simulink model "PubIfDecisionTOS_MDL"  (R2020b)
settings: configuration reference "DspaceConfig" (kept outside this file)
PostLoadFcn:
  | if any(exist('dsrtsu_mdlpostloadfcn', 'file') ~= 0), dsrtsu_mdlpostloadfcn('Execute', bdroot); end
InitFcn:
  | , if any(exist('dsmpb_private', 'file') ~= 0), dsmpb_private('dsmpb_mdlclblib', 'Init', bdroot); end,
undefined symbols (not defined in the file or in its folder): C_TOS_ACCEgoRAxletoFbumplength_m, C_TOS_ACCTargetFront_Flag, C_TOS_AEBJAPedObjDxThre_Val, C_TOS_AEBJAPedObjDyThre_Val, C_TOS_AEBJATargetSize_Val, C_TOS_AEBJAVehObjDxThre_Val, C_TOS_AEBJAVehObjDyThre_Val, C_TOS_AEBJuncPedTargetSize_Val, C_TOS_AEBLatObjDxThre_Val, C_TOS_AEBLatPedDyThre_Val, C_TOS_AEBLatTargetSize_Val, C_TOS_AEBLongTargetInEgoFront_Flag, C_TOS_axAbsGround_Parameter, C_TOS_CameraConfirmedFlag, C_TOS_CNsubjWidth, C_TOS_CurrentLaneCoreMinWidth_Val, C_TOS_CutInProb_Val_Zero, C_TOS_CutOutProb_Val_Zero, C_TOS_D2R_Val, C_TOS_DefaultValueObjectToCenterLine_dy, C_TOS_EgoCarWidth_Val, C_TOS_EgoDxRefPoint_m, C_TOS_EgoRAxletoFbumplength_m, C_TOS_HalfWidthVehicle_Con, C_TOS_HWA_CurrentLaneFlag, C_TOS_HWA_LeftLaneFlag, C_TOS_HWA_MovingDir_Vaild, C_TOS_HWA_MovState_Vaild, C_TOS_HWA_RightLaneFlag, C_TOS_LaneLineCourseErrorFront, C_TOS_LaneLineCourseErrorRear, C_TOS_MotorbikeDefaultWidth_m, C_TOS_NumberOfEffectiveTargets, C_TOS_Obj_Age_Val, C_TOS_Objdx_Constraint_Val, C_TOS_ObjectDefaultWidth_m, C_TOS_ObjInCurrentLane_Val, C_TOS_ObjInCurrentLaneValid, C_TOS_ObjInLeftLaneValid, C_TOS_ObjInRightLaneValid, C_TOS_ObjNotInCurrentLane_Val, C_TOS_ObjNotREElementType, C_TOS_ObjPredictDis_dy_ConstantVal_Zeros, C_TOS_ObjToCenterLine_ConstantVal_Zeros, C_TOS_OFMObjIDInvilad_Val, C_TOS_PIL_LatDisCons_Val_zero, C_TOS_PIL_ObjectCutInFlag_b, C_TOS_PIL_ObjectCutOutFlag_b, C_TOS_PIL_ObjLaneProb_al_Val, C_TOS_PP_ObjFusType_FC_Confirm_b, C_TOS_PP_ObjFusType_FC_FR_Confirm_b, C_TOS_PP_ObjFusType_FR_Confirm_b, C_TOS_RE_80BoolDefault_Val, C_TOS_RE_80Single181Default_Val, C_TOS_RE_80Single255Default_Val, C_TOS_RE_80Uint8Default_Val, C_TOS_RE_D2R, C_TOS_RE_D_180_Val, C_TOS_RE_InvalidObjectID_Val, C_TOS_RE_InvalidTargetChainDir_Val ... (+142)
libraries: simulink x1650, TOS_LIB x361, canfdmsglib x14
(part 33 of 69)

== system PubIfDecisionTOS_MDL/TOS_20201112/TOS_2012080320/PIL_1029/ObjCutInOut_Prob/ObjectCutOut/CutOutProb_Calculate/CutOutProb_Calculate/CutOutPredictDis_dy/CutOutPredictTime_Constraint2 ==
  note: 压线行驶
  note: 目标由右→左；过线
  note: 当前距离dy + 预测距离dy'
  note: 预测距离dy'
  note: 目标由左→右；过线
  ObjectToCenterLine_dy : Inport
  PredictTimeConstraint : Inport  Port=2
  PP_ObjectToCenterLine_vyc : Inport  Port=3
  Object_VY : Inport  Port=4
  Add3 : Sum  OutDataTypeStr=single
  Compare To Constant : simulink/Logic and Bit Operations/Compare To Constant  relop=<  const=C_TOS_ObjToCenterLine_ConstantVal_Zeros  OutDataTypeStr=boolean
      settings: AttributesFormatString=C_TOS_ObjToCenterLine_ConstantVal_Zeros = 0
  Compare To Constant1 : simulink/Logic and Bit Operations/Compare To Constant  relop=>  const=C_TOS_ObjToCenterLine_ConstantVal_Zeros  OutDataTypeStr=boolean
      settings: AttributesFormatString=C_TOS_ObjToCenterLine_ConstantVal_Zeros = 0
  Compare To Constant2 : simulink/Logic and Bit Operations/Compare To Constant  relop=>  const=C_TOS_ObjToCenterLine_ConstantVal_Zeros  OutDataTypeStr=boolean
      settings: AttributesFormatString=C_TOS_ObjToCenterLine_ConstantVal_Zeros = 0
  Compare To Constant3 : simulink/Logic and Bit Operations/Compare To Constant  relop=<  const=C_TOS_ObjToCenterLine_ConstantVal_Zeros  OutDataTypeStr=boolean
      settings: AttributesFormatString=C_TOS_ObjToCenterLine_ConstantVal_Zeros = 0
  Compare To Constant4 : simulink/Logic and Bit Operations/Compare To Constant  relop===  const=C_TOS_ObjToCenterLine_ConstantVal_Zeros  OutDataTypeStr=boolean
      settings: AttributesFormatString=C_TOS_ObjToCenterLine_ConstantVal_Zeros = 0
  Compare To Constant5 : simulink/Logic and Bit Operations/Compare To Constant  relop=>=  const=P_TOS_CutoutObjvyThre  OutDataTypeStr=boolean
      settings: AttributesFormatString=P_TOS_CutoutObjvyThre = 0.3
  Constant : Constant  Value=0  OutDataTypeStr=single
  Constant2 : Constant  Value=C_TOS_ObjPredictDis_dy_ConstantVal_Zeros  OutDataTypeStr=single
      settings: AttributesFormatString=C_TOS_ObjPredictDis_dy_ConstantVal_Zeros = 0
  Constant5 : Constant  Value=C_TOS_ObjPredictDis_dy_ConstantVal_Zeros  OutDataTypeStr=single
      settings: AttributesFormatString=C_TOS_ObjPredictDis_dy_ConstantVal_Zeros = 0
  Constant6 : Constant  Value=C_TOS_ObjPredictDis_dy_ConstantVal_Zeros  OutDataTypeStr=single
      settings: AttributesFormatString=C_TOS_ObjPredictDis_dy_ConstantVal_Zeros = 0
  Divide4 : Product  Inputs=**  OutDataTypeStr=single
  Logical Operator3 : Logic  AllPortsSameDT=off  OutDataTypeStr=boolean
  Logical Operator4 : Logic  AllPortsSameDT=off  OutDataTypeStr=boolean
  Switch : Switch  Criteria=u2 > Threshold
  Switch3 : Switch  Criteria=u2 > Threshold  OutDataTypeStr=single
  Switch4 : Switch  Criteria=u2 > Threshold  OutDataTypeStr=single
  Switch5 : Switch  Criteria=u2 > Threshold  OutDataTypeStr=single
  CutOutPredictDis_dy : Outport  OutDataTypeStr=single
  wires:
  Constant/1 -> Switch/3
  Switch/1 -> Divide4/2
  Compare To Constant5/1 -> Switch/2
  Object_VY/1 -> Compare To Constant5/1
  PP_ObjectToCenterLine_vyc/1 -> Switch/1
  PredictTimeConstraint/1 -> Divide4/1
  Switch4/1 -> Switch3/3
  Compare To Constant2/1 -> Logical Operator4/1
  [ObjectToCenterLine_dy] -> Compare To Constant1/1
  Constant6/1 -> Switch4/1
  Compare To Constant1/1 -> Logical Operator3/2
  Switch5/1 -> Switch4/3
  Constant2/1 -> Switch3/1
  Compare To Constant4/1 -> Switch5/2
  Switch3/1 -> CutOutPredictDis_dy/1
  [ObjectToCenterLine_dy] -> Compare To Constant3/1
  Compare To Constant3/1 -> Logical Operator4/2
  [ObjectToCenterLine_dy] -> Compare To Constant4/1
  ObjectToCenterLine_dy/1 -> Add3/2, [ObjectToCenterLine_dy]
  Divide4/1 -> Add3/1
  Logical Operator4/1 -> Switch4/2
  Add3/1 -> Switch5/3, Compare To Constant2/1, Compare To Constant/1
  Constant5/1 -> Switch5/1
  Logical Operator3/1 -> Switch3/2
  Compare To Constant/1 -> Logical Operator3/1

== system PubIfDecisionTOS_MDL/TOS_20201112/TOS_2012080320/PIL_1029/ObjCutInOut_Prob/ObjectCutOut/CutOutProb_Calculate/CutOutProb_Calculate/CutOutProb/CutOutObjWidthConstraint ==
  note: 根据目标宽度，修正CutOut预测距离（左右车辆边缘）
  note: 目标在中心线左侧
  note: 目标在中心线右侧
  CutOutPredictDis_dy : Inport  OutDataTypeStr=single
  PIL_ObjectToCenterLine_dy_Filt : Inport  Port=2  OutDataTypeStr=single
  Object_Width : Inport  Port=3
  ObjectType : Inport  Port=4
  Add : Sum
  Add1 : Sum  Inputs=+-
  C_HalfWidthVehicle_Con : Constant  Value=C_TOS_HalfWidthVehicle_Con  OutDataTypeStr=single
      settings: AttributesFormatString=C_TOS_HalfWidthVehicle_Con = 0.5
  Constant3 : Constant  Value=C_TOS_ObjToCenterLine_ConstantVal_Zeros  OutDataTypeStr=single
      settings: AttributesFormatString=C_TOS_ObjToCenterLine_ConstantVal_Zeros = 0
  Max : MinMax  Function=max  Inputs=2  OutDataTypeStr=single
  Max1 : MinMax  Inputs=2  OutDataTypeStr=single
  ObjectWidth_Check : Subsystem
  Product : Product  OutDataTypeStr=single
  Relational Operator : RelationalOperator  Operator=>  OutDataTypeStr=boolean  RndMeth=Nearest
  Switch : Switch  Criteria=u2 > Threshold  OutDataTypeStr=single
  constant1 : Constant  Value=0  OutDataTypeStr=single
  constant2 : Constant  Value=0  OutDataTypeStr=single
  CutOutPredictDis_dy_ObjWidthConstraint : Outport
  wires:
  ObjectType/1 -> ObjectWidth_Check/1(ObjectType)
  Object_Width/1 -> ObjectWidth_Check/2(Object_Width)
  ObjectWidth_Check/1(ObjectWidth) -> Product/2
  Add1/1 -> Max1/2
  Product/1 -> Add/1, Add1/2
  C_HalfWidthVehicle_Con/1 -> Product/1
  Relational Operator/1 -> Switch/2
  PIL_ObjectToCenterLine_dy_Filt/1 -> Relational Operator/1
  Constant3/1 -> Relational Operator/2
  constant1/1 -> Max/1
  CutOutPredictDis_dy/1 -> Add/2, Add1/1
  Max/1 -> Switch/1
  constant2/1 -> Max1/1
  Max1/1 -> Switch/3
  Add/1 -> Max/2
  Switch/1 -> CutOutPredictDis_dy_ObjWidthConstraint/1

== system PubIfDecisionTOS_MDL/TOS_20201112/TOS_2012080320/PIL_1029/ObjCutInOut_Prob/ObjectCutOut/CutOutProb_Calculate/CutOutProb_Calculate/CutOutProb/CutOutProb_Calculation ==
  note: 当前值 + 预测值 ；
  note: 预测时机修正
  CutOutPredictDis_dy_ObjWidthConstraint : Inport
  PIL_ObjectToCenterLine_dy_Filt : Inport  Port=2  OutDataTypeStr=single
  Abs : Abs
  Abs1 : Abs
  Add1 : Sum  Inputs=+-  OutDataTypeStr=single
  Add2 : Sum  Inputs=+-  OutDataTypeStr=single
  Compare To Constant1 : simulink/Logic and Bit Operations/Compare To Constant  relop=>=  const=P_TOS_CutOutMaxPredict_dy_Val  OutDataTypeStr=boolean
      settings: AttributesFormatString=P_TOS_CutOutMaxPredict_dy_Val = 2.8
  Compare To Constant2 : simulink/Logic and Bit Operations/Compare To Constant  relop=<=  const=P_TOS_CutOutMinPredict_dy_Val  OutDataTypeStr=boolean
      settings: AttributesFormatString=P_TOS_CutOutMinPredict_dy_Val = 1.5
  Divide1 : Product  Inputs=*/  OutDataTypeStr=single
  K_CutInMaxPredict_dy_Val : Constant  Value=P_TOS_CutOutMaxPredict_dy_Val  OutDataTypeStr=single
      settings: AttributesFormatString=P_TOS_CutOutMaxPredict_dy_Val = 2.8
  K_CutInMaxPredict_dy_Val1 : Constant  Value=P_TOS_CutOutMaxPredict_LatDis_Val  OutDataTypeStr=single
      settings: AttributesFormatString=P_TOS_CutOutMaxPredict_LatDis_Val = 2.8
  K_CutInMinPredict_dy_Val : Constant  Value=P_TOS_CutOutMinPredict_dy_Val  OutDataTypeStr=single
      settings: AttributesFormatString="P_TOS_CutOutMinPredict_dy_Val  = 1.5"
  Relational Operator1 : RelationalOperator  OutDataTypeStr=boolean  RndMeth=Nearest
  Switch1 : Switch  Criteria=u2 > Threshold
  Switch2 : Switch  Criteria=u2 > Threshold
  Switch3 : Switch  Criteria=u2 ~= 0
  CutOutProb_Calculation : Outport
  wires:
  Divide1/1 -> CutOutProb_Calculation/1
  Add2/1 -> Divide1/2
  Add1/1 -> Divide1/1
  [K_CutOutMinPredict_dy_Val] -> Add1/1
  CutOutPredictDis_dy_ObjWidthConstraint/1 -> Abs/1
  Switch2/1 -> Switch1/3
  K_CutInMaxPredict_dy_Val/1 -> [K_CutOutMaxPredict_dy_Val], Switch2/1
  Switch1/1 -> Switch3/3
  [K_CutOutMinPredict_dy_Val] -> Add2/1
  [K_CutOutMaxPredict_dy_Val] -> Add2/2
  K_CutInMinPredict_dy_Val/1 -> Switch1/1, [K_CutOutMinPredict_dy_Val]
  Compare To Constant2/1 -> Switch1/2
  Compare To Constant1/1 -> Switch2/2
  Abs/1 -> Switch2/3, Compare To Constant1/1, Compare To Constant2/1
  PIL_ObjectToCenterLine_dy_Filt/1 -> Abs1/1
  K_CutInMaxPredict_dy_Val1/1 -> Relational Operator1/2
  Relational Operator1/1 -> Switch3/2
  [K_CutOutMinPredict_dy_Val] -> Switch3/1
  Switch3/1 -> Add1/2
  Abs1/1 -> Relational Operator1/1

== system PubIfDecisionTOS_MDL/TOS_20201112/TOS_2012080320/PIL_1029/ObjCutInOut_Prob/ObjectCutOut/CutOutProb_Calculate/CutOutProb_Calculate/CutOutProb_ScopeConstraint/ObjectCutoutMind ==
  PIL_ObjectToCenterLine_dy_Filt : Inport
  PP_ObjectToCenterLine_vyc : Inport  Port=2  OutDataTypeStr=single
  PP_ObjectToCenterLine_dy : Inport  Port=3  OutDataTypeStr=single
  Object_Width : Inport  Port=4
  ObjectType : Inport  Port=5
  Abs1 : Abs
  Abs2 : Abs
  Compare To Constant1 : simulink/Logic and Bit Operations/Compare To Constant  relop=>  const=2.1  OutDataTypeStr=boolean
      settings: AttributesFormatString=P_TOS_CutoutObjvyThre_Val = 0.1
  Compare To Constant2 : simulink/Logic and Bit Operations/Compare To Constant  relop=<=  const=P_TOS_CutoutObjvyThre_Val  OutDataTypeStr=boolean
      settings: AttributesFormatString=P_TOS_CutoutObjvyThre_Val = 0.1
  CutOutObjCutinMov : Subsystem
  CutOutObjWidthConstraint : Subsystem
  Logical Operator1 : Logic  Operator=OR  Inputs=3  AllPortsSameDT=off  OutDataTypeStr=boolean
  Terminator : Terminator
  ObjectCutoutMindFlg : Outport
  ObjectCutoutMindFlg1 : Outport  Port=2
  ObjectCutoutMindFlg2 : Outport  Port=3
  ObjectCutoutMindFlg3 : Outport  Port=4
  wires:
  ObjectType/1 -> CutOutObjWidthConstraint/3(ObjectType)
  Compare To Constant1/1 -> Terminator/1
  Abs2/1 -> Compare To Constant1/1
  PIL_ObjectToCenterLine_dy_Filt/1 -> Abs2/1
  CutOutObjWidthConstraint/1(CutOutPredictDis_dy_ObjWidthConstraint) -> ObjectCutoutMindFlg3/1, Logical Operator1/3
  Logical Operator1/1 -> ObjectCutoutMindFlg/1
  PP_ObjectToCenterLine_dy/1 -> CutOutObjWidthConstraint/1(PP_ObjectToCenterLine_dy), CutOutObjCutinMov/2(ObjectToCenterLine_dy)
  PP_ObjectToCenterLine_vyc/1 -> CutOutObjCutinMov/1(PP_ObjectToCenterLine_vyc), Abs1/1
  Abs1/1 -> Compare To Constant2/1
  Object_Width/1 -> CutOutObjWidthConstraint/2(Object_Width)
  CutOutObjCutinMov/1(CutOutObjCutinMovflg) -> ObjectCutoutMindFlg2/1, Logical Operator1/2
  Compare To Constant2/1 -> ObjectCutoutMindFlg1/1, Logical Operator1/1

== system PubIfDecisionTOS_MDL/TOS_20201112/TOS_2012080320/PIL_1029/ProbCalculat/ProbCalculat/Subsystem/PIL_EgoVehiclePro/EgoVehicle_EgoLaneProb/Data1 ==
  Prob : Inport
  Bus Creator : BusCreator  Inputs=2
  Bus Creator1 : BusCreator  Inputs=2
  Compare To Constant10 : simulink/Logic and Bit Operations/Compare To Constant  relop=>=  const=0.001  OutDataTypeStr=boolean
  Constant1 : Constant  Value=0  OutDataTypeStr=single
  Constant2 : Constant  OutDataTypeStr=uint8
  Constant3 : Constant  Value=0  OutDataTypeStr=uint8
  Switch10 : Switch  Criteria=u2 > Threshold
  Out_Prob1 : Outport
  wires:
  Prob/1 -> Bus Creator/2, Compare To Constant10/1  "Prob1"
  Bus Creator/1 -> Switch10/1
  Bus Creator1/1 -> Switch10/3
  Constant2/1 -> Bus Creator/1  "Count1"
  Switch10/1 -> Out_Prob1/1  "Out_Prob1"
  Constant1/1 -> Bus Creator1/2  "Prob1"
  Constant3/1 -> Bus Creator1/1  "Count1"
  Compare To Constant10/1 -> Switch10/2

== system PubIfDecisionTOS_MDL/TOS_20201112/TOS_2012080320/PIL_1029/ProbCalculat/ProbCalculat/Subsystem/PIL_EgoVehiclePro/EgoVehicle_EgoLaneProb/Data10 ==
  Prob : Inport
  Bus Creator : BusCreator  Inputs=2
  Bus Creator1 : BusCreator  Inputs=2
  Compare To Constant10 : simulink/Logic and Bit Operations/Compare To Constant  relop=>=  const=0.001  OutDataTypeStr=boolean
  Constant1 : Constant  Value=0  OutDataTypeStr=single
  Constant2 : Constant  OutDataTypeStr=uint8
  Constant3 : Constant  Value=0  OutDataTypeStr=uint8
  Switch10 : Switch  Criteria=u2 > Threshold
  Out_Prob10 : Outport
  wires:
  Prob/1 -> Bus Creator/2, Compare To Constant10/1  "Prob10"
  Bus Creator/1 -> Switch10/1
  Bus Creator1/1 -> Switch10/3
  Constant2/1 -> Bus Creator/1  "Count10"
  Switch10/1 -> Out_Prob10/1  "Out_Prob10"
  Constant1/1 -> Bus Creator1/2  "Prob10"
  Constant3/1 -> Bus Creator1/1  "Count10"
  Compare To Constant10/1 -> Switch10/2

== system PubIfDecisionTOS_MDL/TOS_20201112/TOS_2012080320/PIL_1029/ProbCalculat/ProbCalculat/Subsystem/PIL_EgoVehiclePro/EgoVehicle_EgoLaneProb/Data2 ==
  Prob : Inport
  Bus Creator : BusCreator  Inputs=2
  Bus Creator1 : BusCreator  Inputs=2
  Compare To Constant10 : simulink/Logic and Bit Operations/Compare To Constant  relop=>=  const=0.001  OutDataTypeStr=boolean
  Constant1 : Constant  Value=0  OutDataTypeStr=single
  Constant2 : Constant  OutDataTypeStr=uint8
  Constant3 : Constant  Value=0  OutDataTypeStr=uint8
  Switch10 : Switch  Criteria=u2 > Threshold
  Out_Prob2 : Outport
  wires:
  Compare To Constant10/1 -> Switch10/2
  Constant3/1 -> Bus Creator1/1  "Count2"
  Constant1/1 -> Bus Creator1/2  "Prob2"
  Switch10/1 -> Out_Prob2/1  "Out_Prob2"
  Constant2/1 -> Bus Creator/1  "Count2"
  Bus Creator1/1 -> Switch10/3
  Bus Creator/1 -> Switch10/1
  Prob/1 -> Compare To Constant10/1, Bus Creator/2  "Prob2"

== system PubIfDecisionTOS_MDL/TOS_20201112/TOS_2012080320/PIL_1029/ProbCalculat/ProbCalculat/Subsystem/PIL_EgoVehiclePro/EgoVehicle_EgoLaneProb/Data3 ==
  Prob : Inport
  Bus Creator : BusCreator  Inputs=2
  Bus Creator1 : BusCreator  Inputs=2
  Compare To Constant10 : simulink/Logic and Bit Operations/Compare To Constant  relop=>=  const=0.001  OutDataTypeStr=boolean
  Constant1 : Constant  Value=0  OutDataTypeStr=single
  Constant2 : Constant  OutDataTypeStr=uint8
  Constant3 : Constant  Value=0  OutDataTypeStr=uint8
  Switch10 : Switch  Criteria=u2 > Threshold
  Out_Prob3 : Outport
  wires:
  Compare To Constant10/1 -> Switch10/2
  Constant3/1 -> Bus Creator1/1  "Count3"
  Constant1/1 -> Bus Creator1/2  "Prob3"
  Switch10/1 -> Out_Prob3/1  "Out_Prob3"
  Constant2/1 -> Bus Creator/1  "Count3"
  Bus Creator1/1 -> Switch10/3
  Bus Creator/1 -> Switch10/1
  Prob/1 -> Compare To Constant10/1, Bus Creator/2  "Prob3"

== system PubIfDecisionTOS_MDL/TOS_20201112/TOS_2012080320/PIL_1029/ProbCalculat/ProbCalculat/Subsystem/PIL_EgoVehiclePro/EgoVehicle_EgoLaneProb/Data4 ==
  Prob : Inport
  Bus Creator : BusCreator  Inputs=2
  Bus Creator1 : BusCreator  Inputs=2
  Compare To Constant10 : simulink/Logic and Bit Operations/Compare To Constant  relop=>=  const=0.001  OutDataTypeStr=boolean
  Constant1 : Constant  Value=0  OutDataTypeStr=single
  Constant2 : Constant  OutDataTypeStr=uint8
  Constant3 : Constant  Value=0  OutDataTypeStr=uint8
  Switch10 : Switch  Criteria=u2 > Threshold
  Out_Prob4 : Outport
  wires:
  Prob/1 -> Bus Creator/2, Compare To Constant10/1  "Prob4"
  Bus Creator/1 -> Switch10/1
  Bus Creator1/1 -> Switch10/3
  Constant2/1 -> Bus Creator/1  "Count4"
  Switch10/1 -> Out_Prob4/1  "Out_Prob4"
  Constant1/1 -> Bus Creator1/2  "Prob4"
  Constant3/1 -> Bus Creator1/1  "Count4"
  Compare To Constant10/1 -> Switch10/2

== system PubIfDecisionTOS_MDL/TOS_20201112/TOS_2012080320/PIL_1029/ProbCalculat/ProbCalculat/Subsystem/PIL_EgoVehiclePro/EgoVehicle_EgoLaneProb/Data5 ==
  Prob : Inport
  Bus Creator : BusCreator  Inputs=2
  Bus Creator1 : BusCreator  Inputs=2
  Compare To Constant10 : simulink/Logic and Bit Operations/Compare To Constant  relop=>=  const=0.001  OutDataTypeStr=boolean
  Constant1 : Constant  Value=0  OutDataTypeStr=single
  Constant2 : Constant  OutDataTypeStr=uint8
  Constant3 : Constant  Value=0  OutDataTypeStr=uint8
  Switch10 : Switch  Criteria=u2 > Threshold
  Out_Prob5 : Outport
  wires:
  Compare To Constant10/1 -> Switch10/2
  Constant3/1 -> Bus Creator1/1  "Count5"
  Constant1/1 -> Bus Creator1/2  "Prob5"
  Switch10/1 -> Out_Prob5/1  "Out_Prob5"
  Constant2/1 -> Bus Creator/1  "Count5"
  Bus Creator1/1 -> Switch10/3
  Bus Creator/1 -> Switch10/1
  Prob/1 -> Compare To Constant10/1, Bus Creator/2  "Prob5"

== system PubIfDecisionTOS_MDL/TOS_20201112/TOS_2012080320/PIL_1029/ProbCalculat/ProbCalculat/Subsystem/PIL_EgoVehiclePro/EgoVehicle_EgoLaneProb/Data6 ==
  Prob : Inport
  Bus Creator : BusCreator  Inputs=2
  Bus Creator1 : BusCreator  Inputs=2
  Compare To Constant10 : simulink/Logic and Bit Operations/Compare To Constant  relop=>=  const=0.001  OutDataTypeStr=boolean
  Constant1 : Constant  Value=0  OutDataTypeStr=single
  Constant2 : Constant  OutDataTypeStr=uint8
  Constant3 : Constant  Value=0  OutDataTypeStr=uint8
  Switch10 : Switch  Criteria=u2 > Threshold
  Out_Prob6 : Outport
  wires:
  Prob/1 -> Bus Creator/2, Compare To Constant10/1  "Prob6"
  Bus Creator/1 -> Switch10/1
  Bus Creator1/1 -> Switch10/3
  Constant2/1 -> Bus Creator/1  "Count6"
  Switch10/1 -> Out_Prob6/1  "Out_Prob6"
  Constant1/1 -> Bus Creator1/2  "Prob6"
  Constant3/1 -> Bus Creator1/1  "Count6"
  Compare To Constant10/1 -> Switch10/2

== system PubIfDecisionTOS_MDL/TOS_20201112/TOS_2012080320/PIL_1029/ProbCalculat/ProbCalculat/Subsystem/PIL_EgoVehiclePro/EgoVehicle_EgoLaneProb/Data7 ==
  Prob : Inport
  Bus Creator : BusCreator  Inputs=2
  Bus Creator1 : BusCreator  Inputs=2
  Compare To Constant10 : simulink/Logic and Bit Operations/Compare To Constant  relop=>=  const=0.001  OutDataTypeStr=boolean
  Constant1 : Constant  Value=0  OutDataTypeStr=single
  Constant2 : Constant  OutDataTypeStr=uint8
  Constant3 : Constant  Value=0  OutDataTypeStr=uint8
  Switch10 : Switch  Criteria=u2 > Threshold
  Out_Prob7 : Outport
  wires:
  Prob/1 -> Bus Creator/2, Compare To Constant10/1  "Prob7"
  Bus Creator/1 -> Switch10/1
  Bus Creator1/1 -> Switch10/3
  Constant2/1 -> Bus Creator/1  "Count7"
  Switch10/1 -> Out_Prob7/1  "Out_Prob7"
  Constant1/1 -> Bus Creator1/2  "Prob7"
  Constant3/1 -> Bus Creator1/1  "Count7"
  Compare To Constant10/1 -> Switch10/2

== system PubIfDecisionTOS_MDL/TOS_20201112/TOS_2012080320/PIL_1029/ProbCalculat/ProbCalculat/Subsystem/PIL_EgoVehiclePro/EgoVehicle_EgoLaneProb/Data8 ==
  Prob : Inport
  Bus Creator : BusCreator  Inputs=2
  Bus Creator1 : BusCreator  Inputs=2
  Compare To Constant10 : simulink/Logic and Bit Operations/Compare To Constant  relop=>=  const=0.001  OutDataTypeStr=boolean
  Constant1 : Constant  Value=0  OutDataTypeStr=single
  Constant2 : Constant  OutDataTypeStr=uint8
  Constant3 : Constant  Value=0  OutDataTypeStr=uint8
  Switch10 : Switch  Criteria=u2 > Threshold
  Out_Prob8 : Outport
  wires:
  Compare To Constant10/1 -> Switch10/2
  Constant3/1 -> Bus Creator1/1  "Count8"
  Constant1/1 -> Bus Creator1/2  "Prob8"
  Switch10/1 -> Out_Prob8/1  "Out_Prob8"
  Constant2/1 -> Bus Creator/1  "Count8"
  Bus Creator1/1 -> Switch10/3
  Bus Creator/1 -> Switch10/1
  Prob/1 -> Compare To Constant10/1, Bus Creator/2  "Prob8"

== system PubIfDecisionTOS_MDL/TOS_20201112/TOS_2012080320/PIL_1029/ProbCalculat/ProbCalculat/Subsystem/PIL_EgoVehiclePro/EgoVehicle_EgoLaneProb/Data9 ==
  Prob : Inport
  Bus Creator : BusCreator  Inputs=2
  Bus Creator1 : BusCreator  Inputs=2
  Compare To Constant10 : simulink/Logic and Bit Operations/Compare To Constant  relop=>=  const=0.001  OutDataTypeStr=boolean
  Constant1 : Constant  Value=0  OutDataTypeStr=single
  Constant2 : Constant  OutDataTypeStr=uint8
  Constant3 : Constant  Value=0  OutDataTypeStr=uint8
  Switch10 : Switch  Criteria=u2 > Threshold
  Out_Prob9 : Outport
  wires:
  Compare To Constant10/1 -> Switch10/2
  Constant3/1 -> Bus Creator1/1  "Count9"
  Constant1/1 -> Bus Creator1/2  "Prob9"
  Switch10/1 -> Out_Prob9/1  "Out_Prob9"
  Constant2/1 -> Bus Creator/1  "Count9"
  Bus Creator1/1 -> Switch10/3
  Bus Creator/1 -> Switch10/1
  Prob/1 -> Compare To Constant10/1, Bus Creator/2  "Prob9"

== system PubIfDecisionTOS_MDL/TOS_20201112/TOS_2012080320/PIL_1029/ProbCalculat/ProbCalculat/Subsystem/PIL_EgoVehiclePro/EgoVehicle_LeftLaneProb/Data1 ==
  Prob : Inport
  Bus Creator : BusCreator  Inputs=2
  Bus Creator1 : BusCreator  Inputs=2
  Compare To Constant10 : simulink/Logic and Bit Operations/Compare To Constant  relop=>=  const=0.001  OutDataTypeStr=boolean
  Constant1 : Constant  Value=0  OutDataTypeStr=single
  Constant2 : Constant  OutDataTypeStr=uint8
  Constant3 : Constant  Value=0  OutDataTypeStr=uint8
  Switch10 : Switch  Criteria=u2 > Threshold
  Out_Prob1 : Outport
  wires:
  Compare To Constant10/1 -> Switch10/2
  Constant3/1 -> Bus Creator1/1  "Count1"
  Constant1/1 -> Bus Creator1/2  "Prob1"
  Switch10/1 -> Out_Prob1/1  "Out_Prob1"
  Constant2/1 -> Bus Creator/1  "Count1"
  Bus Creator1/1 -> Switch10/3
  Bus Creator/1 -> Switch10/1
  Prob/1 -> Compare To Constant10/1, Bus Creator/2  "Prob1"

== system PubIfDecisionTOS_MDL/TOS_20201112/TOS_2012080320/PIL_1029/ProbCalculat/ProbCalculat/Subsystem/PIL_EgoVehiclePro/EgoVehicle_LeftLaneProb/Data10 ==
  Prob : Inport
  Bus Creator : BusCreator  Inputs=2
  Bus Creator1 : BusCreator  Inputs=2
  Compare To Constant10 : simulink/Logic and Bit Operations/Compare To Constant  relop=>=  const=0.001  OutDataTypeStr=boolean
  Constant1 : Constant  Value=0  OutDataTypeStr=single
  Constant2 : Constant  OutDataTypeStr=uint8
  Constant3 : Constant  Value=0  OutDataTypeStr=uint8
  Switch10 : Switch  Criteria=u2 > Threshold
  Out_Prob10 : Outport
  wires:
  Compare To Constant10/1 -> Switch10/2
  Constant3/1 -> Bus Creator1/1  "Count10"
  Constant1/1 -> Bus Creator1/2  "Prob10"
  Switch10/1 -> Out_Prob10/1  "Out_Prob10"
  Constant2/1 -> Bus Creator/1  "Count10"
  Bus Creator1/1 -> Switch10/3
  Bus Creator/1 -> Switch10/1
  Prob/1 -> Compare To Constant10/1, Bus Creator/2  "Prob10"

== system PubIfDecisionTOS_MDL/TOS_20201112/TOS_2012080320/PIL_1029/ProbCalculat/ProbCalculat/Subsystem/PIL_EgoVehiclePro/EgoVehicle_LeftLaneProb/Data2 ==
  Prob : Inport
  Bus Creator : BusCreator  Inputs=2
  Bus Creator1 : BusCreator  Inputs=2
  Compare To Constant10 : simulink/Logic and Bit Operations/Compare To Constant  relop=>=  const=0.001  OutDataTypeStr=boolean
  Constant1 : Constant  Value=0  OutDataTypeStr=single
  Constant2 : Constant  OutDataTypeStr=uint8
  Constant3 : Constant  Value=0  OutDataTypeStr=uint8
  Switch10 : Switch  Criteria=u2 > Threshold
  Out_Prob2 : Outport
  wires:
  Prob/1 -> Bus Creator/2, Compare To Constant10/1  "Prob2"
  Bus Creator/1 -> Switch10/1
  Bus Creator1/1 -> Switch10/3
  Constant2/1 -> Bus Creator/1  "Count2"
  Switch10/1 -> Out_Prob2/1  "Out_Prob2"
  Constant1/1 -> Bus Creator1/2  "Prob2"
  Constant3/1 -> Bus Creator1/1  "Count2"
  Compare To Constant10/1 -> Switch10/2

== system PubIfDecisionTOS_MDL/TOS_20201112/TOS_2012080320/PIL_1029/ProbCalculat/ProbCalculat/Subsystem/PIL_EgoVehiclePro/EgoVehicle_LeftLaneProb/Data3 ==
  Prob : Inport
  Bus Creator : BusCreator  Inputs=2
  Bus Creator1 : BusCreator  Inputs=2
  Compare To Constant10 : simulink/Logic and Bit Operations/Compare To Constant  relop=>=  const=0.001  OutDataTypeStr=boolean
  Constant1 : Constant  Value=0  OutDataTypeStr=single
  Constant2 : Constant  OutDataTypeStr=uint8
  Constant3 : Constant  Value=0  OutDataTypeStr=uint8
  Switch10 : Switch  Criteria=u2 > Threshold
  Out_Prob3 : Outport
  wires:
  Prob/1 -> Bus Creator/2, Compare To Constant10/1  "Prob3"
  Bus Creator/1 -> Switch10/1
  Bus Creator1/1 -> Switch10/3
  Constant2/1 -> Bus Creator/1  "Count3"
  Switch10/1 -> Out_Prob3/1  "Out_Prob3"
  Constant1/1 -> Bus Creator1/2  "Prob3"
  Constant3/1 -> Bus Creator1/1  "Count3"
  Compare To Constant10/1 -> Switch10/2

== system PubIfDecisionTOS_MDL/TOS_20201112/TOS_2012080320/PIL_1029/ProbCalculat/ProbCalculat/Subsystem/PIL_EgoVehiclePro/EgoVehicle_LeftLaneProb/Data4 ==
  Prob : Inport
  Bus Creator : BusCreator  Inputs=2
  Bus Creator1 : BusCreator  Inputs=2
  Compare To Constant10 : simulink/Logic and Bit Operations/Compare To Constant  relop=>=  const=0.001  OutDataTypeStr=boolean
  Constant1 : Constant  Value=0  OutDataTypeStr=single
  Constant2 : Constant  OutDataTypeStr=uint8
  Constant3 : Constant  Value=0  OutDataTypeStr=uint8
  Switch10 : Switch  Criteria=u2 > Threshold
  Out_Prob4 : Outport
  wires:
  Compare To Constant10/1 -> Switch10/2
  Constant3/1 -> Bus Creator1/1  "Count4"
  Constant1/1 -> Bus Creator1/2  "Prob4"
  Switch10/1 -> Out_Prob4/1  "Out_Prob4"
  Constant2/1 -> Bus Creator/1  "Count4"
  Bus Creator1/1 -> Switch10/3
  Bus Creator/1 -> Switch10/1
  Prob/1 -> Compare To Constant10/1, Bus Creator/2  "Prob4"

== system PubIfDecisionTOS_MDL/TOS_20201112/TOS_2012080320/PIL_1029/ProbCalculat/ProbCalculat/Subsystem/PIL_EgoVehiclePro/EgoVehicle_LeftLaneProb/Data5 ==
  Prob : Inport
  Bus Creator : BusCreator  Inputs=2
  Bus Creator1 : BusCreator  Inputs=2
  Compare To Constant10 : simulink/Logic and Bit Operations/Compare To Constant  relop=>=  const=0.001  OutDataTypeStr=boolean
  Constant1 : Constant  Value=0  OutDataTypeStr=single
  Constant2 : Constant  OutDataTypeStr=uint8
  Constant3 : Constant  Value=0  OutDataTypeStr=uint8
  Switch10 : Switch  Criteria=u2 > Threshold
  Out_Prob5 : Outport
  wires:
  Prob/1 -> Bus Creator/2, Compare To Constant10/1  "Prob5"
  Bus Creator/1 -> Switch10/1
  Bus Creator1/1 -> Switch10/3
  Constant2/1 -> Bus Creator/1  "Count5"
  Switch10/1 -> Out_Prob5/1  "Out_Prob5"
  Constant1/1 -> Bus Creator1/2  "Prob5"
  Constant3/1 -> Bus Creator1/1  "Count5"
  Compare To Constant10/1 -> Switch10/2

== system PubIfDecisionTOS_MDL/TOS_20201112/TOS_2012080320/PIL_1029/ProbCalculat/ProbCalculat/Subsystem/PIL_EgoVehiclePro/EgoVehicle_LeftLaneProb/Data6 ==
  Prob : Inport
  Bus Creator : BusCreator  Inputs=2
  Bus Creator1 : BusCreator  Inputs=2
  Compare To Constant10 : simulink/Logic and Bit Operations/Compare To Constant  relop=>=  const=0.001  OutDataTypeStr=boolean
  Constant1 : Constant  Value=0  OutDataTypeStr=single
  Constant2 : Constant  OutDataTypeStr=uint8
  Constant3 : Constant  Value=0  OutDataTypeStr=uint8
  Switch10 : Switch  Criteria=u2 > Threshold
  Out_Prob6 : Outport
  wires:
  Compare To Constant10/1 -> Switch10/2
  Constant3/1 -> Bus Creator1/1  "Count6"
  Constant1/1 -> Bus Creator1/2  "Prob6"
  Switch10/1 -> Out_Prob6/1  "Out_Prob6"
  Constant2/1 -> Bus Creator/1  "Count6"
  Bus Creator1/1 -> Switch10/3
  Bus Creator/1 -> Switch10/1
  Prob/1 -> Compare To Constant10/1, Bus Creator/2  "Prob6"

== system PubIfDecisionTOS_MDL/TOS_20201112/TOS_2012080320/PIL_1029/ProbCalculat/ProbCalculat/Subsystem/PIL_EgoVehiclePro/EgoVehicle_LeftLaneProb/Data7 ==
  Prob : Inport
  Bus Creator : BusCreator  Inputs=2
  Bus Creator1 : BusCreator  Inputs=2
  Compare To Constant10 : simulink/Logic and Bit Operations/Compare To Constant  relop=>=  const=0.001  OutDataTypeStr=boolean
  Constant1 : Constant  Value=0  OutDataTypeStr=single
  Constant2 : Constant  OutDataTypeStr=uint8
  Constant3 : Constant  Value=0  OutDataTypeStr=uint8
  Switch10 : Switch  Criteria=u2 > Threshold
  Out_Prob7 : Outport
  wires:
  Compare To Constant10/1 -> Switch10/2
  Constant3/1 -> Bus Creator1/1  "Count7"
  Constant1/1 -> Bus Creator1/2  "Prob7"
  Switch10/1 -> Out_Prob7/1  "Out_Prob7"
  Constant2/1 -> Bus Creator/1  "Count7"
  Bus Creator1/1 -> Switch10/3
  Bus Creator/1 -> Switch10/1
  Prob/1 -> Compare To Constant10/1, Bus Creator/2  "Prob7"

== system PubIfDecisionTOS_MDL/TOS_20201112/TOS_2012080320/PIL_1029/ProbCalculat/ProbCalculat/Subsystem/PIL_EgoVehiclePro/EgoVehicle_LeftLaneProb/Data8 ==
  Prob : Inport
  Bus Creator : BusCreator  Inputs=2
  Bus Creator1 : BusCreator  Inputs=2
  Compare To Constant10 : simulink/Logic and Bit Operations/Compare To Constant  relop=>=  const=0.001  OutDataTypeStr=boolean
  Constant1 : Constant  Value=0  OutDataTypeStr=single
  Constant2 : Constant  OutDataTypeStr=uint8
  Constant3 : Constant  Value=0  OutDataTypeStr=uint8
  Switch10 : Switch  Criteria=u2 > Threshold
  Out_Prob8 : Outport
  wires:
  Prob/1 -> Bus Creator/2, Compare To Constant10/1  "Prob8"
  Bus Creator/1 -> Switch10/1
  Bus Creator1/1 -> Switch10/3
  Constant2/1 -> Bus Creator/1  "Count8"
  Switch10/1 -> Out_Prob8/1  "Out_Prob8"
  Constant1/1 -> Bus Creator1/2  "Prob8"
  Constant3/1 -> Bus Creator1/1  "Count8"
  Compare To Constant10/1 -> Switch10/2

== system PubIfDecisionTOS_MDL/TOS_20201112/TOS_2012080320/PIL_1029/ProbCalculat/ProbCalculat/Subsystem/PIL_EgoVehiclePro/EgoVehicle_LeftLaneProb/Data9 ==
  Prob : Inport
  Bus Creator : BusCreator  Inputs=2
  Bus Creator1 : BusCreator  Inputs=2
  Compare To Constant10 : simulink/Logic and Bit Operations/Compare To Constant  relop=>=  const=0.001  OutDataTypeStr=boolean
  Constant1 : Constant  Value=0  OutDataTypeStr=single
  Constant2 : Constant  OutDataTypeStr=uint8
  Constant3 : Constant  Value=0  OutDataTypeStr=uint8
  Switch10 : Switch  Criteria=u2 > Threshold
  Out_Prob9 : Outport
  wires:
  Prob/1 -> Bus Creator/2, Compare To Constant10/1  "Prob9"
  Bus Creator/1 -> Switch10/1
  Bus Creator1/1 -> Switch10/3
  Constant2/1 -> Bus Creator/1  "Count9"
  Switch10/1 -> Out_Prob9/1  "Out_Prob9"
  Constant1/1 -> Bus Creator1/2  "Prob9"
  Constant3/1 -> Bus Creator1/1  "Count9"
  Compare To Constant10/1 -> Switch10/2

== system PubIfDecisionTOS_MDL/TOS_20201112/TOS_2012080320/PIL_1029/ProbCalculat/ProbCalculat/Subsystem/PIL_EgoVehiclePro/EgoVehicle_RightLaneProb/Data1 ==
  Prob : Inport
  Bus Creator : BusCreator  Inputs=2
  Bus Creator1 : BusCreator  Inputs=2
  Compare To Constant10 : simulink/Logic and Bit Operations/Compare To Constant  relop=>=  const=0.001  OutDataTypeStr=boolean
  Constant1 : Constant  Value=0  OutDataTypeStr=single
  Constant2 : Constant  OutDataTypeStr=uint8
  Constant3 : Constant  Value=0  OutDataTypeStr=uint8
  Switch10 : Switch  Criteria=u2 > Threshold
  Out_Prob1 : Outport
  wires:
  Compare To Constant10/1 -> Switch10/2
  Constant3/1 -> Bus Creator1/1  "Count1"
  Constant1/1 -> Bus Creator1/2  "Prob1"
  Switch10/1 -> Out_Prob1/1  "Out_Prob1"
  Constant2/1 -> Bus Creator/1  "Count1"
  Bus Creator1/1 -> Switch10/3
  Bus Creator/1 -> Switch10/1
  Prob/1 -> Compare To Constant10/1, Bus Creator/2  "Prob1"

== system PubIfDecisionTOS_MDL/TOS_20201112/TOS_2012080320/PIL_1029/ProbCalculat/ProbCalculat/Subsystem/PIL_EgoVehiclePro/EgoVehicle_RightLaneProb/Data10 ==
  Prob : Inport
  Bus Creator : BusCreator  Inputs=2
  Bus Creator1 : BusCreator  Inputs=2
  Compare To Constant10 : simulink/Logic and Bit Operations/Compare To Constant  relop=>=  const=0.001  OutDataTypeStr=boolean
  Constant1 : Constant  Value=0  OutDataTypeStr=single
  Constant2 : Constant  OutDataTypeStr=uint8
  Constant3 : Constant  Value=0  OutDataTypeStr=uint8
  Switch10 : Switch  Criteria=u2 > Threshold
  Out_Prob10 : Outport
  wires:
  Compare To Constant10/1 -> Switch10/2
  Constant3/1 -> Bus Creator1/1  "Count10"
  Constant1/1 -> Bus Creator1/2  "Prob10"
  Switch10/1 -> Out_Prob10/1  "Out_Prob10"
  Constant2/1 -> Bus Creator/1  "Count10"
  Bus Creator1/1 -> Switch10/3
  Bus Creator/1 -> Switch10/1
  Prob/1 -> Compare To Constant10/1, Bus Creator/2  "Prob10"

== system PubIfDecisionTOS_MDL/TOS_20201112/TOS_2012080320/PIL_1029/ProbCalculat/ProbCalculat/Subsystem/PIL_EgoVehiclePro/EgoVehicle_RightLaneProb/Data2 ==
  Prob : Inport
  Bus Creator : BusCreator  Inputs=2
  Bus Creator1 : BusCreator  Inputs=2
  Compare To Constant10 : simulink/Logic and Bit Operations/Compare To Constant  relop=>=  const=0.001  OutDataTypeStr=boolean
  Constant1 : Constant  Value=0  OutDataTypeStr=single
  Constant2 : Constant  OutDataTypeStr=uint8
  Constant3 : Constant  Value=0  OutDataTypeStr=uint8
  Switch10 : Switch  Criteria=u2 > Threshold
  Out_Prob2 : Outport
  wires:
  Prob/1 -> Bus Creator/2, Compare To Constant10/1  "Prob2"
  Bus Creator/1 -> Switch10/1
  Bus Creator1/1 -> Switch10/3
  Constant2/1 -> Bus Creator/1  "Count2"
  Switch10/1 -> Out_Prob2/1  "Out_Prob2"
  Constant1/1 -> Bus Creator1/2  "Prob2"
  Constant3/1 -> Bus Creator1/1  "Count2"
  Compare To Constant10/1 -> Switch10/2

== system PubIfDecisionTOS_MDL/TOS_20201112/TOS_2012080320/PIL_1029/ProbCalculat/ProbCalculat/Subsystem/PIL_EgoVehiclePro/EgoVehicle_RightLaneProb/Data3 ==
  Prob : Inport
  Bus Creator : BusCreator  Inputs=2
  Bus Creator1 : BusCreator  Inputs=2
  Compare To Constant10 : simulink/Logic and Bit Operations/Compare To Constant  relop=>=  const=0.001  OutDataTypeStr=boolean
  Constant1 : Constant  Value=0  OutDataTypeStr=single
  Constant2 : Constant  OutDataTypeStr=uint8
  Constant3 : Constant  Value=0  OutDataTypeStr=uint8
  Switch10 : Switch  Criteria=u2 > Threshold
  Out_Prob3 : Outport
  wires:
  Prob/1 -> Bus Creator/2, Compare To Constant10/1  "Prob3"
  Bus Creator/1 -> Switch10/1
  Bus Creator1/1 -> Switch10/3
  Constant2/1 -> Bus Creator/1  "Count3"
  Switch10/1 -> Out_Prob3/1  "Out_Prob3"
  Constant1/1 -> Bus Creator1/2  "Prob3"
  Constant3/1 -> Bus Creator1/1  "Count3"
  Compare To Constant10/1 -> Switch10/2

== system PubIfDecisionTOS_MDL/TOS_20201112/TOS_2012080320/PIL_1029/ProbCalculat/ProbCalculat/Subsystem/PIL_EgoVehiclePro/EgoVehicle_RightLaneProb/Data4 ==
  Prob : Inport
  Bus Creator : BusCreator  Inputs=2
  Bus Creator1 : BusCreator  Inputs=2
  Compare To Constant10 : simulink/Logic and Bit Operations/Compare To Constant  relop=>=  const=0.001  OutDataTypeStr=boolean
  Constant1 : Constant  Value=0  OutDataTypeStr=single
  Constant2 : Constant  OutDataTypeStr=uint8
  Constant3 : Constant  Value=0  OutDataTypeStr=uint8
  Switch10 : Switch  Criteria=u2 > Threshold
  Out_Prob4 : Outport
  wires:
  Compare To Constant10/1 -> Switch10/2
  Constant3/1 -> Bus Creator1/1  "Count4"
  Constant1/1 -> Bus Creator1/2  "Prob4"
  Switch10/1 -> Out_Prob4/1  "Out_Prob4"
  Constant2/1 -> Bus Creator/1  "Count4"
  Bus Creator1/1 -> Switch10/3
  Bus Creator/1 -> Switch10/1
  Prob/1 -> Compare To Constant10/1, Bus Creator/2  "Prob4"

== system PubIfDecisionTOS_MDL/TOS_20201112/TOS_2012080320/PIL_1029/ProbCalculat/ProbCalculat/Subsystem/PIL_EgoVehiclePro/EgoVehicle_RightLaneProb/Data5 ==
  Prob : Inport
  Bus Creator : BusCreator  Inputs=2
  Bus Creator1 : BusCreator  Inputs=2
  Compare To Constant10 : simulink/Logic and Bit Operations/Compare To Constant  relop=>=  const=0.001  OutDataTypeStr=boolean
  Constant1 : Constant  Value=0  OutDataTypeStr=single
  Constant2 : Constant  OutDataTypeStr=uint8
  Constant3 : Constant  Value=0  OutDataTypeStr=uint8
  Switch10 : Switch  Criteria=u2 > Threshold
  Out_Prob5 : Outport
  wires:
  Prob/1 -> Bus Creator/2, Compare To Constant10/1  "Prob5"
  Bus Creator/1 -> Switch10/1
  Bus Creator1/1 -> Switch10/3
  Constant2/1 -> Bus Creator/1  "Count5"
  Switch10/1 -> Out_Prob5/1  "Out_Prob5"
  Constant1/1 -> Bus Creator1/2  "Prob5"
  Constant3/1 -> Bus Creator1/1  "Count5"
  Compare To Constant10/1 -> Switch10/2

== system PubIfDecisionTOS_MDL/TOS_20201112/TOS_2012080320/PIL_1029/ProbCalculat/ProbCalculat/Subsystem/PIL_EgoVehiclePro/EgoVehicle_RightLaneProb/Data6 ==
  Prob : Inport
  Bus Creator : BusCreator  Inputs=2
  Bus Creator1 : BusCreator  Inputs=2
  Compare To Constant10 : simulink/Logic and Bit Operations/Compare To Constant  relop=>=  const=0.001  OutDataTypeStr=boolean
  Constant1 : Constant  Value=0  OutDataTypeStr=single
  Constant2 : Constant  OutDataTypeStr=uint8
  Constant3 : Constant  Value=0  OutDataTypeStr=uint8
  Switch10 : Switch  Criteria=u2 > Threshold
  Out_Prob6 : Outport
  wires:
  Compare To Constant10/1 -> Switch10/2
  Constant3/1 -> Bus Creator1/1  "Count6"
  Constant1/1 -> Bus Creator1/2  "Prob6"
  Switch10/1 -> Out_Prob6/1  "Out_Prob6"
  Constant2/1 -> Bus Creator/1  "Count6"
  Bus Creator1/1 -> Switch10/3
  Bus Creator/1 -> Switch10/1
  Prob/1 -> Compare To Constant10/1, Bus Creator/2  "Prob6"

== system PubIfDecisionTOS_MDL/TOS_20201112/TOS_2012080320/PIL_1029/ProbCalculat/ProbCalculat/Subsystem/PIL_EgoVehiclePro/EgoVehicle_RightLaneProb/Data7 ==
  Prob : Inport
  Bus Creator : BusCreator  Inputs=2
  Bus Creator1 : BusCreator  Inputs=2
  Compare To Constant10 : simulink/Logic and Bit Operations/Compare To Constant  relop=>=  const=0.001  OutDataTypeStr=boolean
  Constant1 : Constant  Value=0  OutDataTypeStr=single
  Constant2 : Constant  OutDataTypeStr=uint8
  Constant3 : Constant  Value=0  OutDataTypeStr=uint8
  Switch10 : Switch  Criteria=u2 > Threshold
  Out_Prob7 : Outport
  wires:
  Compare To Constant10/1 -> Switch10/2
  Constant3/1 -> Bus Creator1/1  "Count7"
  Constant1/1 -> Bus Creator1/2  "Prob7"
  Switch10/1 -> Out_Prob7/1  "Out_Prob7"
  Constant2/1 -> Bus Creator/1  "Count7"
  Bus Creator1/1 -> Switch10/3
  Bus Creator/1 -> Switch10/1
  Prob/1 -> Compare To Constant10/1, Bus Creator/2  "Prob7"

== system PubIfDecisionTOS_MDL/TOS_20201112/TOS_2012080320/PIL_1029/ProbCalculat/ProbCalculat/Subsystem/PIL_EgoVehiclePro/EgoVehicle_RightLaneProb/Data8 ==
  Prob : Inport
  Bus Creator : BusCreator  Inputs=2
  Bus Creator1 : BusCreator  Inputs=2
  Compare To Constant10 : simulink/Logic and Bit Operations/Compare To Constant  relop=>=  const=0.001  OutDataTypeStr=boolean
  Constant1 : Constant  Value=0  OutDataTypeStr=single
  Constant2 : Constant  OutDataTypeStr=uint8
  Constant3 : Constant  Value=0  OutDataTypeStr=uint8
  Switch10 : Switch  Criteria=u2 > Threshold
  Out_Prob8 : Outport
  wires:
  Prob/1 -> Bus Creator/2, Compare To Constant10/1  "Prob8"
  Bus Creator/1 -> Switch10/1
  Bus Creator1/1 -> Switch10/3
  Constant2/1 -> Bus Creator/1  "Count8"
  Switch10/1 -> Out_Prob8/1  "Out_Prob8"
  Constant1/1 -> Bus Creator1/2  "Prob8"
  Constant3/1 -> Bus Creator1/1  "Count8"
  Compare To Constant10/1 -> Switch10/2

== system PubIfDecisionTOS_MDL/TOS_20201112/TOS_2012080320/PIL_1029/ProbCalculat/ProbCalculat/Subsystem/PIL_EgoVehiclePro/EgoVehicle_RightLaneProb/Data9 ==
  Prob : Inport
  Bus Creator : BusCreator  Inputs=2
  Bus Creator1 : BusCreator  Inputs=2
  Compare To Constant10 : simulink/Logic and Bit Operations/Compare To Constant  relop=>=  const=0.001  OutDataTypeStr=boolean
  Constant1 : Constant  Value=0  OutDataTypeStr=single
  Constant2 : Constant  OutDataTypeStr=uint8
  Constant3 : Constant  Value=0  OutDataTypeStr=uint8
  Switch10 : Switch  Criteria=u2 > Threshold
  Out_Prob9 : Outport
  wires:
  Prob/1 -> Bus Creator/2, Compare To Constant10/1  "Prob9"
  Bus Creator/1 -> Switch10/1
  Bus Creator1/1 -> Switch10/3
  Constant2/1 -> Bus Creator/1  "Count9"
  Switch10/1 -> Out_Prob9/1  "Out_Prob9"
  Constant1/1 -> Bus Creator1/2  "Prob9"
  Constant3/1 -> Bus Creator1/1  "Count9"
  Compare To Constant10/1 -> Switch10/2

== system PubIfDecisionTOS_MDL/TOS_20201112/TOS_2012080320/PP1128/AAT-AdditionalAttributes/PP_ObjectToCenterLine_dy/PP_EgoVeh_Object_ToCenterLine/PP_ObjectToCenterLine/PP_ObjectToCenterLine_/line01_DisJudge ==
  Object_DX : Inport
  line01_dDisStart : Inport  Port=2
  line01_dDisEnd : Inport  Port=3
  Logical Operator : Logic  AllPortsSameDT=off  OutDataTypeStr=boolean
  Relational Operator : RelationalOperator  OutDataTypeStr=boolean  RndMeth=Nearest
  Relational Operator1 : RelationalOperator  Operator=<  OutDataTypeStr=boolean  RndMeth=Nearest
  line01_DisJudge : Outport
  wires:
  line01_dDisEnd/1 -> Relational Operator1/2
  line01_dDisStart/1 -> Relational Operator/2
  Object_DX/1 -> Relational Operator1/1, Relational Operator/1
  Relational Operator/1 -> Logical Operator/1
  Relational Operator1/1 -> Logical Operator/2
  Logical Operator/1 -> line01_DisJudge/1

== system PubIfDecisionTOS_MDL/TOS_20201112/TOS_2012080320/PP1128/AAT-AdditionalAttributes/PP_ObjectToCenterLine_dy/PP_EgoVeh_Object_ToCenterLine/PP_ObjectToCenterLine/PP_ObjectToCenterLine_/line01_dy ==
  Object_DX : Inport
  line01_C0 : Inport  Port=2
  line01_C1 : Inport  Port=3
  line01_C2 : Inport  Port=4
  line01_C3 : Inport  Port=5
  Add : Sum
  Add1 : Sum
  Add3 : Sum
  Constant1 : Constant  Value=3  OutDataTypeStr=single
  Math Function1 : Math  Operator=pow  SignedPower=on  SaturateOnIntegerOverflow=on
  Product : Product
  Product1 : Product
  Product2 : Product
  Square : Math  Operator=square  SignedPower=on  SaturateOnIntegerOverflow=on
  line01_dy : Outport
  wires:
  line01_C1/1 -> Product1/2
  line01_C3/1 -> Product2/2
  Add3/1 -> line01_dy/1
  Add/1 -> Add3/1
  Constant1/1 -> Math Function1/2
  Product1/1 -> Add1/2
  Product2/1 -> Add3/2
  Math Function1/1 -> Product2/1
  Object_DX/1 -> Math Function1/1, Square/1, Product1/1
  Square/1 -> Product/1
  line01_C2/1 -> Product/2
  Product/1 -> Add/2
  line01_C0/1 -> Add1/1
  Add1/1 -> Add/1

== system PubIfDecisionTOS_MDL/TOS_20201112/TOS_2012080320/PP1128/AAT-AdditionalAttributes/PP_ObjectToCenterLine_dy/PP_EgoVeh_Object_ToCenterLine/PP_ObjectToCenterLine/PP_ObjectToCenterLine_/line02_DisJudge ==
  Object_DX : Inport
  line02_dDisStart : Inport  Port=2
  line02_dDisEnd : Inport  Port=3
  Logical Operator : Logic  AllPortsSameDT=off  OutDataTypeStr=boolean
  Relational Operator : RelationalOperator  OutDataTypeStr=boolean  RndMeth=Nearest
  Relational Operator1 : RelationalOperator  Operator=<  OutDataTypeStr=boolean  RndMeth=Nearest
  line02_DisJudge : Outport
  wires:
  Logical Operator/1 -> line02_DisJudge/1
  Relational Operator1/1 -> Logical Operator/2
  Relational Operator/1 -> Logical Operator/1
  Object_DX/1 -> Relational Operator/1, Relational Operator1/1
  line02_dDisStart/1 -> Relational Operator/2
  line02_dDisEnd/1 -> Relational Operator1/2

== system PubIfDecisionTOS_MDL/TOS_20201112/TOS_2012080320/PP1128/AAT-AdditionalAttributes/PP_ObjectToCenterLine_dy/PP_EgoVeh_Object_ToCenterLine/PP_ObjectToCenterLine/PP_ObjectToCenterLine_/line02_dy ==
  Object_DX : Inport
  line02_C0 : Inport  Port=2
  line02_C1 : Inport  Port=3
  line02_C2 : Inport  Port=4
  line02_C3 : Inport  Port=5
  Add : Sum
  Add1 : Sum
  Add3 : Sum
  Constant1 : Constant  Value=3  OutDataTypeStr=single
  Math Function1 : Math  Operator=pow  SignedPower=on  SaturateOnIntegerOverflow=on
  Product : Product
  Product1 : Product
  Product2 : Product
  Square : Math  Operator=square  SignedPower=on  SaturateOnIntegerOverflow=on
  line02_dy : Outport
  wires:
  Add1/1 -> Add/1
  line02_C0/1 -> Add1/1
  Product/1 -> Add/2
  line02_C2/1 -> Product/2
  Square/1 -> Product/1
  Object_DX/1 -> Product1/1, Square/1, Math Function1/1
  Math Function1/1 -> Product2/1
  Product2/1 -> Add3/2
  Product1/1 -> Add1/2
  Constant1/1 -> Math Function1/2
  Add/1 -> Add3/1
  Add3/1 -> line02_dy/1
  line02_C3/1 -> Product2/2
  line02_C1/1 -> Product1/2

== system PubIfDecisionTOS_MDL/TOS_20201112/TOS_2012080320/PP1128/AAT-AdditionalAttributes/PP_ObjectToCenterLine_dy/PP_EgoVeh_Object_ToCenterLine/PP_ObjectToCenterLine/PP_ObjectToCenterLine_/line03_DisJudge ==
  Object_DX : Inport
  line03_dDisStart : Inport  Port=2
  line03_dDisEnd : Inport  Port=3
  Logical Operator : Logic  AllPortsSameDT=off  OutDataTypeStr=boolean
  Relational Operator : RelationalOperator  OutDataTypeStr=boolean  RndMeth=Nearest
  Relational Operator1 : RelationalOperator  Operator=<  OutDataTypeStr=boolean  RndMeth=Nearest
  line03_DisJudge : Outport
  wires:
  line03_dDisEnd/1 -> Relational Operator1/2
  line03_dDisStart/1 -> Relational Operator/2
  Object_DX/1 -> Relational Operator1/1, Relational Operator/1
  Relational Operator/1 -> Logical Operator/1
  Relational Operator1/1 -> Logical Operator/2
  Logical Operator/1 -> line03_DisJudge/1

== system PubIfDecisionTOS_MDL/TOS_20201112/TOS_2012080320/PP1128/AAT-AdditionalAttributes/PP_ObjectToCenterLine_dy/PP_EgoVeh_Object_ToCenterLine/PP_ObjectToCenterLine/PP_ObjectToCenterLine_/line03_dy ==
  Object_DX : Inport
  line03_C0 : Inport  Port=2
  line03_C1 : Inport  Port=3
  line03_C2 : Inport  Port=4
  line03_C3 : Inport  Port=5
  Add : Sum
  Add1 : Sum
  Add3 : Sum
  Constant1 : Constant  Value=3  OutDataTypeStr=single
  Math Function1 : Math  Operator=pow  SignedPower=on  SaturateOnIntegerOverflow=on
  Product : Product
  Product1 : Product
  Product2 : Product
  Square : Math  Operator=square  SignedPower=on  SaturateOnIntegerOverflow=on
  line03_dy : Outport
  wires:
  line03_C1/1 -> Product1/2
  line03_C3/1 -> Product2/2
  Add3/1 -> line03_dy/1
  Add/1 -> Add3/1
  Constant1/1 -> Math Function1/2
  Product1/1 -> Add1/2
  Product2/1 -> Add3/2
  Math Function1/1 -> Product2/1
  Object_DX/1 -> Math Function1/1, Square/1, Product1/1
  Square/1 -> Product/1
  line03_C2/1 -> Product/2
  Product/1 -> Add/2
  line03_C0/1 -> Add1/1
  Add1/1 -> Add/1

== system PubIfDecisionTOS_MDL/TOS_20201112/TOS_2012080320/PP1128/AAT-AdditionalAttributes/PP_ObjectToCenterLine_dy/PP_EgoVeh_Object_ToCenterLine/PP_ObjectToCenterLine/PP_ObjectToCenterLine_/line04_DisJudge ==
  Object_DX : Inport
  line04_dDisStart : Inport  Port=2
  line04_dDisEnd : Inport  Port=3
  Logical Operator : Logic  AllPortsSameDT=off  OutDataTypeStr=boolean
  Relational Operator : RelationalOperator  OutDataTypeStr=boolean  RndMeth=Nearest
  Relational Operator1 : RelationalOperator  Operator=<  OutDataTypeStr=boolean  RndMeth=Nearest
  line04_DisJudge : Outport
  wires:
  Logical Operator/1 -> line04_DisJudge/1
  Relational Operator1/1 -> Logical Operator/2
  Relational Operator/1 -> Logical Operator/1
  Object_DX/1 -> Relational Operator/1, Relational Operator1/1
  line04_dDisStart/1 -> Relational Operator/2
  line04_dDisEnd/1 -> Relational Operator1/2

== system PubIfDecisionTOS_MDL/TOS_20201112/TOS_2012080320/PP1128/AAT-AdditionalAttributes/PP_ObjectToCenterLine_dy/PP_EgoVeh_Object_ToCenterLine/PP_ObjectToCenterLine/PP_ObjectToCenterLine_/line04_dy ==
  Object_DX : Inport
  line04_C0 : Inport  Port=2
  line04_C1 : Inport  Port=3
  line04_C2 : Inport  Port=4
  line04_C3 : Inport  Port=5
  Add : Sum
  Add1 : Sum
  Add3 : Sum
  Constant1 : Constant  Value=3  OutDataTypeStr=single
  Math Function1 : Math  Operator=pow  SignedPower=on  SaturateOnIntegerOverflow=on
  Product : Product
  Product1 : Product
  Product2 : Product
  Square : Math  Operator=square  SignedPower=on  SaturateOnIntegerOverflow=on
  line04_dy : Outport
  wires:
  Add1/1 -> Add/1
  line04_C0/1 -> Add1/1
  Product/1 -> Add/2
  line04_C2/1 -> Product/2
  Square/1 -> Product/1
  Object_DX/1 -> Product1/1, Square/1, Math Function1/1
  Math Function1/1 -> Product2/1
  Product2/1 -> Add3/2
  Product1/1 -> Add1/2
  Constant1/1 -> Math Function1/2
  Add/1 -> Add3/1
  Add3/1 -> line04_dy/1
  line04_C3/1 -> Product2/2
  line04_C1/1 -> Product1/2

== system PubIfDecisionTOS_MDL/TOS_20201112/TOS_2012080320/PP1128/AAT-AdditionalAttributes/PP_ObjectToCenterLine_dy/PP_EgoVeh_Object_ToCenterLine/PP_ObjectToCenterLine/PP_ObjectToCenterLine_/line05_DisJudge ==
  Object_DX : Inport
  line05_dDisStart : Inport  Port=2
  line05_dDisEnd : Inport  Port=3
  Logical Operator : Logic  AllPortsSameDT=off  OutDataTypeStr=boolean
  Relational Operator : RelationalOperator  OutDataTypeStr=boolean  RndMeth=Nearest
  Relational Operator1 : RelationalOperator  Operator=<  OutDataTypeStr=boolean  RndMeth=Nearest
  line05_DisJudge : Outport
  wires:
  line05_dDisEnd/1 -> Relational Operator1/2
  line05_dDisStart/1 -> Relational Operator/2
  Object_DX/1 -> Relational Operator1/1, Relational Operator/1
  Relational Operator/1 -> Logical Operator/1
  Relational Operator1/1 -> Logical Operator/2
  Logical Operator/1 -> line05_DisJudge/1
